simulink model "lab3sim"  (R2022b)
settings: Solver=ode5  StartTime=0.0  StopTime=120.0s  RelTol=1e-3
values from neighbouring files (symbols this model uses):
  g = 9.81    [lab3simcode.m]
  h = 1.70 * 0.547    (= 0.9299)    [lab3simcode.m]
  I = 1.70^2 * 65.77 * 0.547    (= 103.9711891)    [lab3simcode.m]
  m = 65.77 * 0.971    (= 63.86267)    [lab3simcode.m]
  Tau_e = 0.04    [lab3simcode.m]
  Tau_f = 0.01    [lab3simcode.m]
  Tau_m = 0.05    [lab3simcode.m]
undefined symbols (not defined in the file or in its folder): Kd, Kp
settings Model: Creator=irwin  LastModifiedBy=irwin

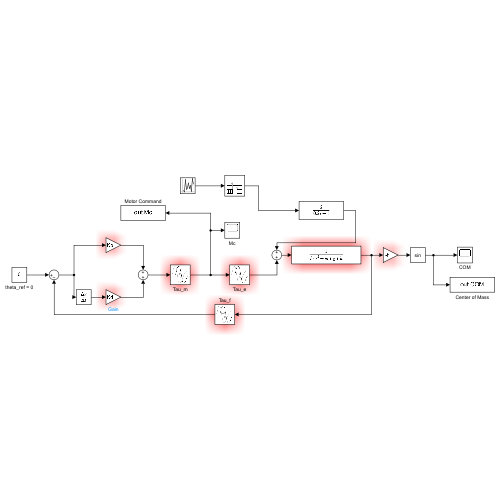
[thumbnail: Simulink's stored preview of the top-level diagram]
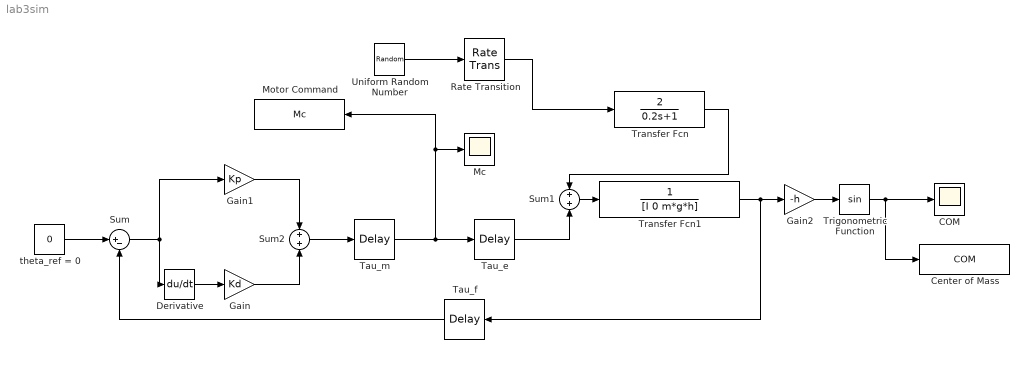
== system lab3sim ==
  COM : Scope
  Center of Mass : ToWorkspace  VariableName=COM  SampleTime=-1
  Derivative : Derivative
  Gain : Gain  Gain=Kd
  Gain1 : Gain  Gain=Kp
  Gain2 : Gain  Gain=-h
  Mc : Scope
  Motor Command : ToWorkspace  VariableName=Mc  SampleTime=-1
  Rate Transition : RateTransition
  Sum : Sum  Inputs=|+-
  Sum1 : Sum
  Sum2 : Sum
  Tau_e : TransportDelay  DelayTime=Tau_e
  Tau_f : TransportDelay  DelayTime=Tau_f
  Tau_m : TransportDelay  DelayTime=Tau_m
  Transfer Fcn : TransferFcn  Numerator=[2]  Denominator=[0.2 1]
  Transfer Fcn1 : TransferFcn  Denominator=[I 0 m*g*h]
  Trigonometric Function : Trigonometry
  Uniform Random Number : UniformRandomNumber  Minimum=-4  Maximum=4  SampleTime=0.1
  theta_ref = 0 : Constant  Value=0
  wires:
  theta_ref = 0/1 -> Sum/1
  Derivative/1 -> Gain/1
  Sum/1 -> Derivative/1, Gain1/1
  Gain/1 -> Sum2/2
  Gain1/1 -> Sum2/1
  Sum2/1 -> Tau_m/1
  Tau_m/1 -> Motor Command/1, Mc/1, Tau_e/1
  Uniform Random Number/1 -> Rate Transition/1
  Tau_e/1 -> Sum1/2
  Transfer Fcn/1 -> Sum1/1
  Rate Transition/1 -> Transfer Fcn/1
  Sum1/1 -> Transfer Fcn1/1
  Transfer Fcn1/1 -> Tau_f/1, Gain2/1
  Tau_f/1 -> Sum/2
  Trigonometric Function/1 -> Center of Mass/1, COM/1
  Gain2/1 -> Trigonometric Function/1
